simulink model "wolnozmienny_interpolacja"  (R2017b)
settings: Solver=FixedStepDiscrete  StartTime=0.0  StopTime=0.0  RelTol=1e-3
undefined symbols (not defined in the file): H, W
libraries: CPOiS_SourcesSinks x8, CPOiS_DataManipulation x3
settings Model: Creator=alis  LastModifiedBy=alis

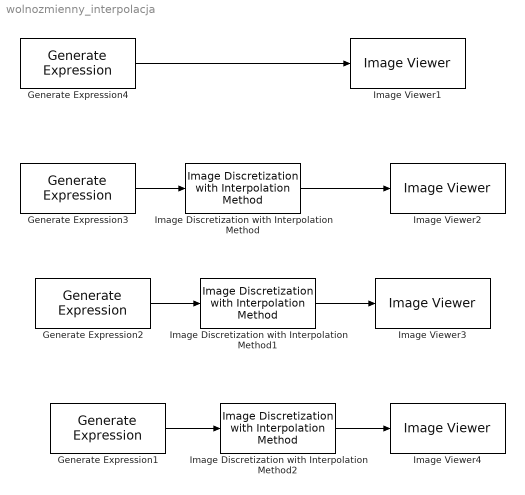
== system wolnozmienny_interpolacja ==
  Generate Expression{1..4} (4 alike) : CPOiS_SourcesSinks/Generate Expression  Width=256  Height=256  Expression=W/2+H/2
      settings: SourceProductName=CPOiS - Digital image and signal processing
  Image Discretization with Interpolation Method : CPOiS_DataManipulation/Image Discretization with Interpolation Method  factor=8  method=nearest
      settings: SourceProductName=CPOiS - Digital image and signal processing
  Image Discretization with Interpolation Method1 : CPOiS_DataManipulation/Image Discretization with Interpolation Method  factor=8  method=bilinear
      settings: SourceProductName=CPOiS - Digital image and signal processing
  Image Discretization with Interpolation Method2 : CPOiS_DataManipulation/Image Discretization with Interpolation Method  factor=8  method=bicubic
      settings: SourceProductName=CPOiS - Digital image and signal processing
  Image Viewer{1..4} (4 alike) : CPOiS_SourcesSinks/Image Viewer
      settings: SourceProductName=CPOiS - Digital image and signal processing
  wires:
  Generate Expression4/1 -> Image Viewer1/1
  Image Discretization with Interpolation Method/1 -> Image Viewer2/1
  Generate Expression3/1 -> Image Discretization with Interpolation Method/1
  Image Discretization with Interpolation Method1/1 -> Image Viewer3/1
  Generate Expression2/1 -> Image Discretization with Interpolation Method1/1
  Image Discretization with Interpolation Method2/1 -> Image Viewer4/1
  Generate Expression1/1 -> Image Discretization with Interpolation Method2/1
